simulink model "AdaptiveCompTorque"  (R2019b)
settings: Solver=ode45  StartTime=0.0  StopTime=50
undefined symbols (not defined in the file): a0, a1, a2, a3, B, dq0, Kd_endEff, Kp_endEff, P, parameter, Pi, Pi0, q0, R, x_endEff_D
libraries: cstblocks x1, simulink x1
settings Model: Creator=ariannagasparri  LastModifiedBy=ariannagasparri

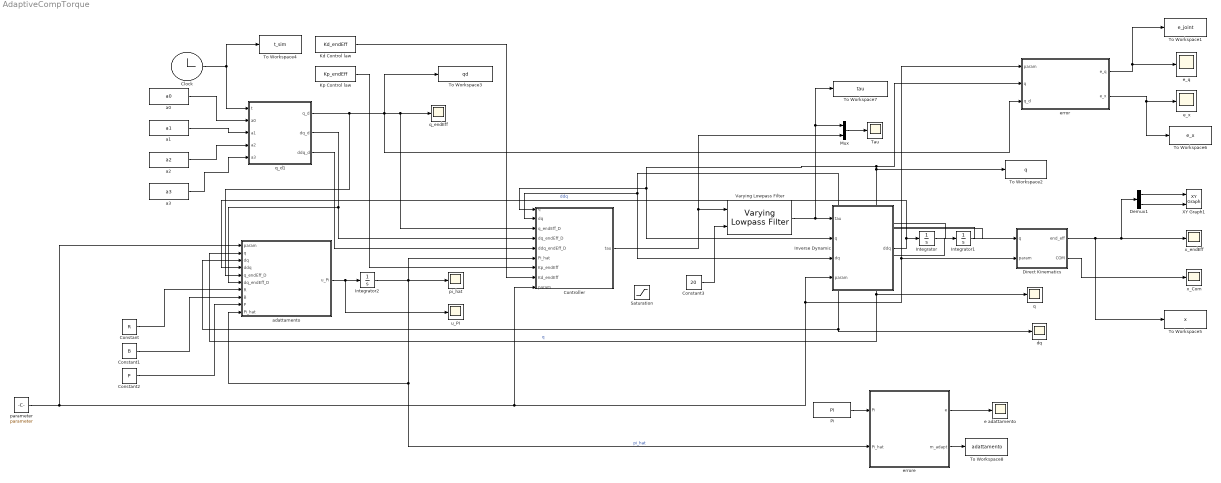
== system AdaptiveCompTorque ==
  Clock : Clock
  Constant : Constant  Value=R
  Constant1 : Constant  Value=B
  Constant2 : Constant  Value=P
  Constant3 : Constant  Value=20
  Controller : MATLAB Function  TreatAsAtomicUnit=on
  Demux1 : Demux  Outputs=3
  "Direct Kinematics " : MATLAB Function  TreatAsAtomicUnit=on
  Integrator : Integrator  InitialCondition=dq0
  Integrator1 : Integrator  InitialCondition=q0
  Integrator2 : Integrator  InitialCondition=Pi0
  "Inverse Dynamic " : MATLAB Function  TreatAsAtomicUnit=on
  Kd Control law : Constant  Value=Kd_endEff
  Kp Control law : Constant  Value=Kp_endEff
  Mux : Mux  Inputs=2
  Pi : Constant  Value=Pi
  Saturation : Saturate  UpperLimit=1500  LowerLimit=-1500
  Tau : Scope
  To Workspace1 : ToWorkspace  VariableName=e_joint  SaveFormat=Structure With Time  SampleTime=-1
  To Workspace2 : ToWorkspace  VariableName=q  SaveFormat=Structure With Time  SampleTime=-1
  To Workspace3 : ToWorkspace  VariableName=qd  SaveFormat=Structure With Time  SampleTime=-1
  To Workspace4 : ToWorkspace  VariableName=t_sim  SaveFormat=Structure With Time  SampleTime=-1
  To Workspace5 : ToWorkspace  VariableName=x  SaveFormat=Structure With Time  SampleTime=-1
  To Workspace6 : ToWorkspace  VariableName=e_x  SaveFormat=Structure With Time  SampleTime=-1
  To Workspace7 : ToWorkspace  VariableName=tau  SaveFormat=Structure With Time  SampleTime=-1
  To Workspace8 : ToWorkspace  VariableName=adattamento  SaveFormat=Structure With Time  SampleTime=-1
  Varying Lowpass Filter : cstblocks/Linear Parameter Varying/Varying Lowpass Filter  N=1
      settings: SourceProductName=Control System Toolbox
  XY Graph1 : simulink/Sinks/XY Graph  xmin=x_endEff_D(1)-2  xmax=x_endEff_D(1)+2  ymin=x_endEff_D(3)-2  ymax=x_endEff_D(3)+2  st=-1
  a0 : Constant  Value=a0
  a1 : Constant  Value=a1
  a2 : Constant  Value=a2
  a3 : Constant  Value=a3
  adattamento : MATLAB Function  TreatAsAtomicUnit=on
  dq : Scope
  e adattamento : Scope
  e_q : Scope
  e_x : Scope
  error : MATLAB Function  TreatAsAtomicUnit=on
  errore : MATLAB Function  TreatAsAtomicUnit=on
  "parameter " : Constant  Value=parameter
  pi_hat : Scope
  q : Scope
  q_d1 : MATLAB Function  TreatAsAtomicUnit=on
  q_endEff : Scope
  u_PI : Scope
  x_Com : Scope
  x_endEff : Scope
  wires:
  Integrator/1 -> adattamento/3(dq), dq/1, Integrator1/1, "Inverse Dynamic "/3(dq), Controller/2(dq)
  adattamento/1(u_Pi) -> u_PI/1, Integrator2/1
  Integrator2/1 -> Controller/6(Pi_hat), pi_hat/1, errore/2(Pi_hat), adattamento/10(Pi_hat)  "pi_hat"
  Integrator1/1 -> "Inverse Dynamic "/2(q), Controller/1(q), error/2(q), To Workspace2/1, "Direct Kinematics "/1(q), adattamento/2(q), q/1  "q"
  "Inverse Dynamic "/1(ddq) -> Integrator/1, adattamento/4(ddq)  "ddq"
  a3/1 -> q_d1/5(a3)
  q_d1/2(dq_d) -> adattamento/6(dq_endEff_D), Controller/4(dq_endEff_D)
  a0/1 -> q_d1/2(a0)
  q_d1/3(ddq_d) -> Controller/5(ddq_endEff_D)
  Clock/1 -> q_d1/1(t), To Workspace4/1
  a1/1 -> q_d1/3(a1)
  a2/1 -> q_d1/4(a2)
  "Direct Kinematics "/2(COM) -> x_Com/1
  Demux1/1 -> XY Graph1/1
  Demux1/3 -> XY Graph1/2
  "Direct Kinematics "/1(end_eff) -> To Workspace5/1, Demux1/1, x_endEff/1
  "parameter "/1 -> "Direct Kinematics "/2(param), error/1(param), "Inverse Dynamic "/4(param), Controller/9(param), adattamento/1(param)
  q_d1/1(q_d) -> adattamento/5(q_endEff_D), error/3(q_d), Controller/3(q_endEff_D), q_endEff/1, To Workspace3/1
  error/2(e_x) -> To Workspace6/1, e_x/1
  error/1(e_q) -> To Workspace1/1, e_q/1
  Kp Control law/1 -> Controller/7(Kp_endEff)
  Kd Control law/1 -> Controller/8(Kd_endEff)
  Constant/1 -> adattamento/7(R)
  Constant1/1 -> adattamento/8(B)
  Constant2/1 -> adattamento/9(P)
  errore/1(e) -> e adattamento/1
  errore/2(m_adapt) -> To Workspace8/1
  Pi/1 -> errore/1(Pi)
  Varying Lowpass Filter/1 -> Mux/1, To Workspace7/1, "Inverse Dynamic "/1(tau)
  Constant3/1 -> Varying Lowpass Filter/2
  Mux/1 -> Tau/1
  Controller/1(tau) -> Mux/2, Varying Lowpass Filter/1

== matlab function AdaptiveCompTorque/errore ==
  data: Pi input; Pi_hat input; e output; m_adapt output
function [e, m_adapt]  = ErroreAdattamento(Pi, Pi_hat)
    
    e = Pi - Pi_hat;
    
    m_adapt = [Pi_hat(1,1), Pi_hat(2,1), Pi_hat(3,1), Pi_hat(4,1), Pi_hat(5,1), Pi_hat(6,1)]';

end

== matlab function AdaptiveCompTorque/Controller ==
  data: q input; dq input; q_endEff_D input; dq_endEff_D input; ddq_endEff_D input; Pi_hat input; Kp_endEff input; Kd_endEff input; tau output; param input
function tau  = x_now(q, dq, q_endEff_D, dq_endEff_D, ddq_endEff_D, Pi_hat, Kp_endEff, Kd_endEff, param)

% ddq, 
%     Y = Y_fun(param, q, dq, ddq);
    Y = Y_fun(param, q, dq, ddq_endEff_D); 

    %% controllo Diretto
    
    e_endEff = q_endEff_D - q;
    de_endEff = dq_endEff_D - dq;
    
    tau = Y*Pi_hat + Kp_endEff*e_endEff + Kd_endEff*de_endEff;

end

== matlab function AdaptiveCompTorque/adattamento ==
  data: param input; q input; dq input; ddq input; u_Pi output; q_endEff_D input; dq_endEff_D input; R input; B input; P input; Pi_hat input
function u_Pi = Adattamento(param, q, dq, ddq, q_endEff_D, dq_endEff_D, R, B, P, Pi_hat)

    m_hat = [Pi_hat(1), Pi_hat(2),Pi_hat(3), Pi_hat(4), Pi_hat(5), Pi_hat(6)]';
    param_hat = [param(:,1), m_hat, param(:,3)];
    
    %param è corretto qui perchè tanto Y_fun non 
    %è funzione dei parametri da adattare.
    Y = Y_fun(param, q, dq, ddq);
    
    M_hat = B_fun(param_hat, q);

    e_endEff = q_endEff_D - q;
    de_endEff = dq_endEff_D - dq;
    x = [e_endEff; de_endEff];

    u_Pi = inv(R) * Y' * (inv(M_hat))' * B' * P * x;
end

== matlab function AdaptiveCompTorque/Inverse Dynamic  ==
  data: tau input size=[6,1]; q input size=[6,1]; dq input size=[6,1]; ddq output size=[6,1]; param input
function ddq = inverseDynamic(tau,q,dq,param)

    B = B_fun(param, q);
    C = C_fun(param, q, dq);
    G = G_fun(param, q);

    ddq = B\(tau - G - C*dq);

end

== matlab function AdaptiveCompTorque/Direct Kinematics  ==
  data: q input; end_eff output; param input; COM output
function [end_eff, COM] = DirectK(q,param)


    [Pcom, Etip,T00,T01,T12,T23,T34,T45,T56] =  forwardKinematics(param, q);
    
    
    end_eff = Etip(1:3,4);
    COM = Pcom;
    
end

== matlab function AdaptiveCompTorque/q_d1 ==
  data: t input; q_d output; dq_d output; ddq_d output; a0 input; a1 input; a2 input; a3 input
function [q_d,dq_d,ddq_d] = desiderable_q(t, a0,a1,a2,a3)

    [q_d, dq_d, ddq_d] = vettoreq(a0,a1,a2,a3,t);
    
end

== matlab function AdaptiveCompTorque/error ==
  data: param input; q input; e_q output; q_d input; e_x output
function [e_q, e_x]  = error(param, q, q_d)
    

%     [~, Etip,~,~,~,~,~,~,~] =  forwardKinematics(param, q*pi/180);
%     [~, Etip_d,~,~,~,~,~,~,~] =  forwardKinematics(param, q_d*pi/180);  

    [~, Etip,~,~,~,~,~,~,~] =  forwardKinematics(param, q);
    [~, Etip_d,~,~,~,~,~,~,~] =  forwardKinematics(param, q_d);  

    e_x = Etip_d(1:3,4) - Etip(1:3,4);

    e_q = q_d - q;
    
end
